simulink model "uncontrolled_group24"  (R2023b)
settings: Solver=ode5  StartTime=0.0  StopTime=333  FixedStep=0.1  RelTol=1e-3
values from neighbouring files (symbols this model uses):
  a = 6939    [Air_Drag_script.m]    (also in main.m = 6939.063; main_group24.m = 6939.063)
  A0 = eye(3)    [Air_Drag_script.m]    (also in main_group24.m)
  ARW = 0.15    [main_group24.m]
  c = 2.99792*10^8    (= 299792000)    [main.m]    (also in main_group24.m)
  e = 0    [Air_Drag_script.m]    (also in main.m = 0.001304; main_group24.m)
  G = [gn, gm, gvali, gsvi]    [main.m]    (also in main_group24.m)
  GyroSampleRate = 10    [main_group24.m]
  H = [hn, hm, hvali, hsvi]    [main.m]    (also in main_group24.m)
  i = deg2rad(97.5307)    [Air_Drag_script.m]    (also in main.m; main_group24.m)
  I_tot = [Ix 0 0; 0 Iy 0; 0 0 Iz]    [data_mass.m]    (also in main_group24.m)
  invI_tot = inv(I_tot)    [data_mass.m]    (also in main_group24.m)
  Ix = J(1,1)    [Air_Drag_script.m]    (also in data_mass.m = 0.0755003333333; main.m = 0.057749855; main_group24.m = 0.0755003333333)
  Iy = J(2,2)    [Air_Drag_script.m]    (also in data_mass.m = 0.0755003333333; main.m = 0.04143542; main_group24.m = 0.0755003333333)
  Iz = J(3,3)    [Air_Drag_script.m]    (also in data_mass.m = 0.055; main.m = 0.024624309; main_group24.m = 0.055)
  m = [0.1; 0.1; 0.1]    [main.m]    (also in main_group24.m)
  MB = [4; 0.1; 0.1; 0.3]    [main.m]    (also in main_group24.m)
  MMnoise = 15e-9*[1; 1; 1]    [main_group24.m]
  MMSampleRate = 1    [main_group24.m]
  mu = 3.98600433e+5    (= 398600.433)    [main.m]    (also in main_group24.m)
  n = 0.0011    [Air_Drag_script.m]    (also in main.m = sqrt(mu/a^3); main_group24.m = sqrt(mu/a^3))
  q0 = [ 1 1 1 1 ]'    [Air_Drag_script.m]    (also in main_group24.m = [0 0 0 1]')
  R_e = 6378    [main.m]    (also in main_group24.m)
  rho_air = 1.65e-13    [Air_Drag_script.m]
  rho_d_MB = 0.1    [main.m]    (also in main_group24.m)
  rho_d_SP = 0.1    [main.m]    (also in main_group24.m)
  rho_s_MB = 0.5    [main.m]    (also in main_group24.m)
  rho_s_SP = 0.1    [main.m]    (also in main_group24.m)
  RRW = 0.3    [main_group24.m]
  SP = [1; 0.3; 0.1; 0.01]    [main.m]    (also in main_group24.m = [0.25; 0.1; 0.3; 0.01])
  w0 = [0 0 0]'    [Air_Drag_script.m]    (also in main.m = [wx0; wy0; wz0]; main_group24.m = [wx0; wy0; wz0])
undefined symbols (not defined in the file or in its folder): Cd, H_0, n_E, P, pan1, pan2, rho_d_body, rho_d_sp, rho_s_body, rho_s_sp, s1, s2, s3, s4, s5, s6, v_rel
libraries: vrlib x40, simulink_extras x13, matrix_library x8, sharedutil x3, simulink x1
(part 1 of 4)
settings Model: Creator=lucag  LastModifiedBy=lucag
settings OptimizationCC: ReuseModelBlockBuffer=off

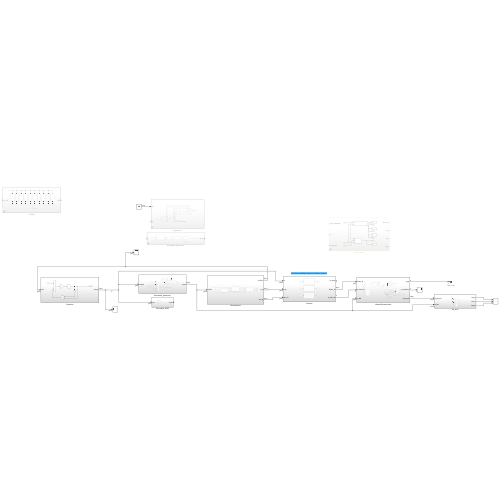
[thumbnail: Simulink's stored preview of the top-level diagram]
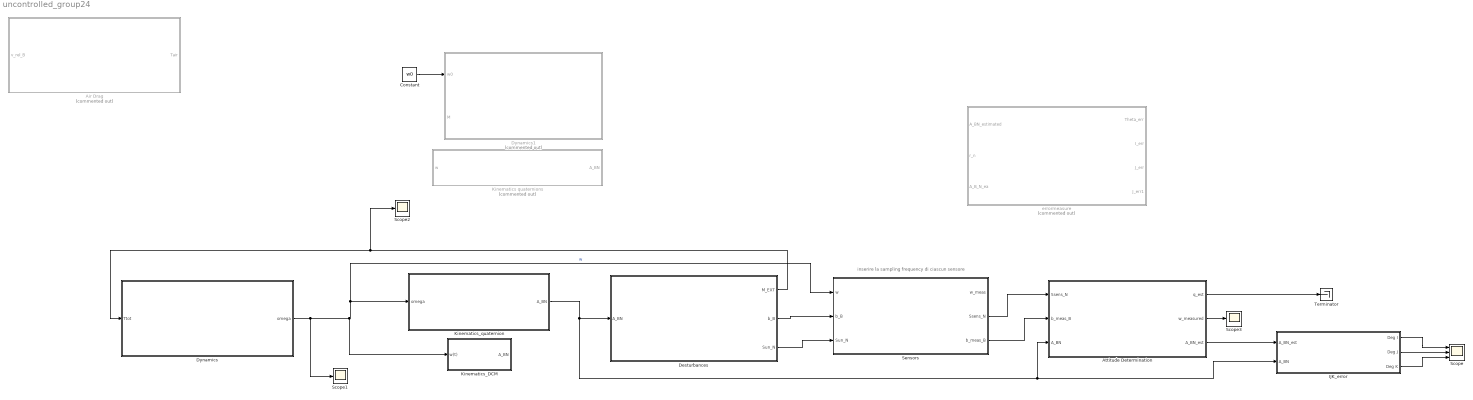
== system uncontrolled_group24 ==
  note: inserire la sampling frequency di ciascun sensore
  Air Drag : Subsystem  Commented=on
  Attitude Determination : Subsystem
  Constant : Constant  Value=w0  VectorParams1D=off
  Desturbances : Subsystem
  Dynamics : Subsystem
  Dynamics1 : Subsystem  Commented=on
  IJK_error : Subsystem
  Kinematics quaternions : Subsystem  Commented=on
  Kinematics_DCM : Subsystem
  Kinematics_quaternion : Subsystem
  Scope : Scope  NumInputPorts=3
  Scope1 : Scope
  Scope2 : Scope
  Scope3 : Scope
  Sensors : Subsystem
  Terminator : Terminator
  errormeasure : Subsystem  Commented=on
  wires:
  Desturbances/2(b_B) -> Sensors/2(b_B)
  Desturbances/3(Sun_N) -> Sensors/3(Sun_N)
  Sensors/3(b_meas_B) -> Attitude Determination/2(b_meas_B)
  Constant/1 -> Dynamics1/1(w0)
  Sensors/2(Ssens_N) -> Attitude Determination/1(Ssens_N)
  Dynamics/1(omega) -> Scope1/1, Kinematics_DCM/1(w(t)), Kinematics_quaternion/1(omega), Sensors/1(w)  "w"
  Attitude Determination/1(q_est) -> Terminator/1
  Desturbances/1(M_EXT) -> Dynamics/1(Ttot), Scope2/1
  Attitude Determination/2(w_measured) -> Scope3/1
  Kinematics_quaternion/1(A_BN) -> Attitude Determination/3(A_BN), IJK_error/2(A_BN), Desturbances/1(A_BN)
  Attitude Determination/3(A_BN_est) -> IJK_error/1(A_BN_est)
  IJK_error/2(Deg J) -> Scope/2
  IJK_error/1(Deg I) -> Scope/1
  IJK_error/3(Deg K) -> Scope/3

== system uncontrolled_group24/Air Drag ==
  v_rel_B : Inport
  Subsystem : Subsystem
  Subsystem1 : Subsystem
  Subsystem2 : Subsystem
  Subsystem3 : Subsystem
  Subsystem4 : Subsystem
  Subsystem5 : Subsystem
  Subsystem6 : Subsystem
  Subsystem7 : Subsystem
  Subsystem8 : Subsystem
  Subsystem9 : Subsystem
  Sum : Sum  Inputs=++++++++++
  Tair : Outport
  wires:
  v_rel_B/1 -> Subsystem1/1(v_rel_B), Subsystem2/1(v_rel_B), Subsystem3/1(v_rel_B), Subsystem4/1(v_rel_B), Subsystem5/1(v_rel_B), Subsystem6/1(v_rel_B), Subsystem7/1(v_rel_B), Subsystem8/1(v_rel_B), Subsystem9/1(v_rel_B), Subsystem/1(v_rel_B)
  Sum/1 -> Tair/1
  Subsystem/1(Pan1) -> Sum/1
  Subsystem1/1(Pan2) -> Sum/2
  Subsystem2/1(Pan3) -> Sum/3
  Subsystem3/1(Pan4) -> Sum/4
  Subsystem4/1(Pan5) -> Sum/5
  Subsystem5/1(Pan6) -> Sum/6
  Subsystem6/1(Ps1) -> Sum/7
  Subsystem7/1(Ps2) -> Sum/8
  Subsystem8/1(Ps3) -> Sum/9
  Subsystem9/1(Ps4) -> Sum/10

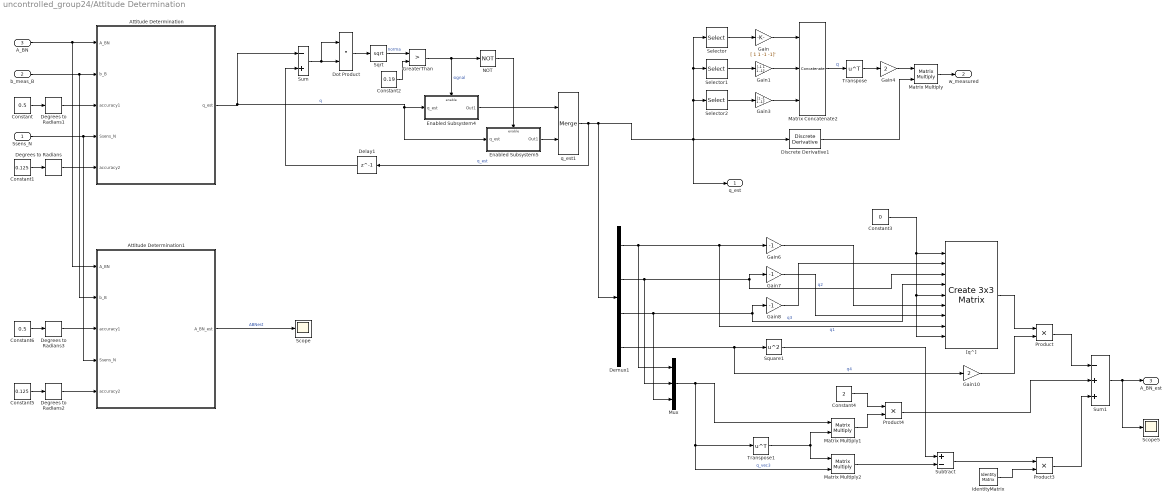
== system uncontrolled_group24/Attitude Determination ==
  Ssens_N : Inport
  b_meas_B : Inport  Port=2
  A_BN : Inport  Port=3
  Attitude Determination : MATLAB Function  TreatAsAtomicUnit=on
  Attitude Determination1 : MATLAB Function  TreatAsAtomicUnit=on
  Constant : Constant  Value=0.5
  Constant1 : Constant  Value=0.125
  Constant2 : Constant  Value=0.19
  Constant3 : Constant  Value=0
  Constant4 : Constant  Value=2
  Constant5 : Constant  Value=0.125
  Constant6 : Constant  Value=0.5
  Degrees to Radians{,1..3} (4 alike) : simulink_extras/Transformations/Degrees to Radians
  Delay1 : Delay  DelayLength=1  InitialCondition=q0
  Demux1 : Demux
  Discrete Derivative1 : simulink/Discrete/Discrete Derivative  gainval=1.0  ICPrevScaledInput=0  OutMin=[]  OutMax=[]  OutDataType=fixdt(1, 16)  OutScaling=2^-10  DoSatur=off
  Dot Product : DotProduct  OutDataTypeStr=Inherit: Inherit via internal rule
  Enabled Subsystem4 : Subsystem  TreatAsAtomicUnit=on
  Enabled Subsystem5 : Subsystem  TreatAsAtomicUnit=on
  Gain : Gain  Gain=[ 1 1 -1 -1]'
  Gain1 : Gain  Gain=[-1 1 1 -1]'
  Gain10 : Gain  Gain=2
  Gain3 : Gain  Gain=[1 -1 1 -1]'
  Gain4 : Gain  Gain=2
  Gain6 : Gain  Gain=-1
  Gain7 : Gain  Gain=-1
  Gain8 : Gain  Gain=-1
  GreaterThan : RelationalOperator  Operator=>  OutDataTypeStr=boolean  RndMeth=Simplest  InputSameDT=off
  IdentityMatrix : IdentityMatrix  OutputDimensions=3
  Matrix Concatenate2 : Concatenate  NumInputs=3  Mode=Multidimensional array  ConcatenateDimension=2
  Matrix Multiply : Product  Multiplication=Matrix(*)
  Matrix Multiply1 : Product  Multiplication=Matrix(*)
  Matrix Multiply2 : Product  Multiplication=Matrix(*)
  Mux : Mux  Inputs=3
  NOT : Logic  Operator=NOT  IconShape=distinctive  AllPortsSameDT=off  OutDataTypeStr=boolean
  Product : Product
  Product3 : Product
  Product4 : Product
  Scope : Scope
  Scope5 : Scope
  Selector : Selector  InputPortWidth=4  IndexOptions=Index vector (dialog)  Indices=[4 3 2 1]  OutputSizes=1
  Selector1 : Selector  InputPortWidth=4  IndexOptions=Index vector (dialog)  Indices=[3 4 1 2]  OutputSizes=1
  Selector2 : Selector  InputPortWidth=4  IndexOptions=Index vector (dialog)  Indices=[2 1 4 3]  OutputSizes=1
  Sqrt : Sqrt
  Square1 : Math  Operator=square
  Subtract : Sum  Inputs=+-
  Sum : Sum  Inputs=-+
  Sum1 : Sum  Inputs=-++
  Transpose : Math  Operator=transpose
  Transpose1 : Math  Operator=transpose
  "[q^]" : sharedutil/Create 3x3 Matrix  aMode=aMode
      settings: LibrarySourceBlock=aerolibutil/Create 3x3 Matrix
  q_est1 : Merge
  q_est : Outport
  w_measured : Outport  Port=2
  A_BN_est : Outport  Port=3
  wires:
  b_meas_B/1 -> Attitude Determination1/2(b_B), Attitude Determination/2(b_B)
  Ssens_N/1 -> Attitude Determination1/4(Ssens_N), Attitude Determination/4(Ssens_N)
  Constant1/1 -> Degrees to Radians/1
  Constant/1 -> Degrees to Radians1/1
  A_BN/1 -> Attitude Determination1/1(A_BN), Attitude Determination/1(A_BN)
  Gain1/1 -> Matrix Concatenate2/2
  Matrix Multiply/1 -> w_measured/1
  Gain4/1 -> Matrix Multiply/1
  Gain/1 -> Matrix Concatenate2/1
  Selector/1 -> Gain/1
  Selector2/1 -> Gain3/1
  Transpose/1 -> Gain4/1
  Discrete Derivative1/1 -> Matrix Multiply/2
  Matrix Concatenate2/1 -> Transpose/1  "Q"
  Selector1/1 -> Gain1/1
  Gain3/1 -> Matrix Concatenate2/3
  Degrees to Radians1/1 -> Attitude Determination/3(accuracy1)
  Degrees to Radians/1 -> Attitude Determination/5(accuracy2)
  q_est1/1 -> Demux1/1, q_est/1, Selector1/1, Selector/1, Selector2/1, Discrete Derivative1/1, Delay1/1  "q_est"
  GreaterThan/1 -> NOT/1, Enabled Subsystem4/Enable  "signal"
  Enabled Subsystem5/1(Out1) -> q_est1/2
  Sum/1 -> Dot Product/1, Dot Product/2
  Delay1/1 -> Sum/2
  NOT/1 -> Enabled Subsystem5/Enable
  Enabled Subsystem4/1(Out1) -> q_est1/1
  Constant2/1 -> GreaterThan/2
  Sqrt/1 -> GreaterThan/1  "norma"
  Dot Product/1 -> Sqrt/1
  Attitude Determination/1(q_est) -> Enabled Subsystem4/1(q_est), Enabled Subsystem5/1(q_est), Sum/1  "q"
  "[q^]"/1 -> Product/1
  Square1/1 -> Subtract/1
  Matrix Multiply1/1 -> Product4/2
  Gain10/1 -> Product/2
  Sum1/1 -> Scope5/1, A_BN_est/1
  Product/1 -> Sum1/1
  Gain8/1 -> "[q^]"/2
  Constant4/1 -> Product4/1
  Mux/1 -> Matrix Multiply1/1, Transpose1/1, Matrix Multiply2/2  "q_vec3"
  IdentityMatrix/1 -> Product3/2
  Transpose1/1 -> Matrix Multiply1/2, Matrix Multiply2/1
  Matrix Multiply2/1 -> Subtract/2
  Demux1/4 -> Gain10/1, Square1/1  "q4"
  Gain6/1 -> "[q^]"/6
  Demux1/2 -> Mux/2, Gain7/1, "[q^]"/3  "q2"
  Constant3/1 -> "[q^]"/5, "[q^]"/9, "[q^]"/1
  Gain7/1 -> "[q^]"/7
  Demux1/3 -> Mux/3, Gain8/1, "[q^]"/4  "q3"
  Product3/1 -> Sum1/3
  Product4/1 -> Sum1/2
  Demux1/1 -> Mux/1, Gain6/1, "[q^]"/8  "q1"
  Subtract/1 -> Product3/1
  Attitude Determination1/1(A_BN_est) -> Scope/1  "ABNest"
  Degrees to Radians2/1 -> Attitude Determination1/5(accuracy2)
  Constant5/1 -> Degrees to Radians2/1
  Degrees to Radians3/1 -> Attitude Determination1/3(accuracy1)
  Constant6/1 -> Degrees to Radians3/1

== system uncontrolled_group24/Desturbances ==
  A_BN : Inport
  External Torques : Subsystem
  Orbital Mechanics : Subsystem
  Relative Attitude : Subsystem
  M_EXT : Outport
  b_B : Outport  Port=2
  Sun_N : Outport  Port=3
  wires:
  Relative Attitude/1(A_BL.) -> External Torques/1(A_BL)
  Relative Attitude/2(r_L) -> External Torques/2(r_L)
  A_BN/1 -> External Torques/4(A_BN), Relative Attitude/1(A_BN_ideal)
  Orbital Mechanics/1(theta) -> Relative Attitude/2(theta)
  Orbital Mechanics/2(r_N) -> Relative Attitude/3(r_N)
  Orbital Mechanics/3(r) -> External Torques/3(r)
  External Torques/1(M_EXT) -> M_EXT/1
  External Torques/2(b_B) -> b_B/1
  External Torques/3(Sun_N) -> Sun_N/1

== system uncontrolled_group24/Dynamics ==
  note: omega
  Ttot : Inport
  Add : Sum
  Cross Product : vrlib/Utilities/Cross Product
  Gain : Gain  Gain=invI_tot  Multiplication=Matrix(K*u)
  Gain1 : Gain  Gain=I_tot  Multiplication=Matrix(K*u)
  Integrator3 : Integrator  InitialCondition=w0  AbsoluteTolerance=10^-7
  omega : Outport
  wires:
  Gain1/1 -> Cross Product/1
  Ttot/1 -> Add/1
  Cross Product/1 -> Add/2
  Integrator3/1 -> omega/1, Cross Product/2, Gain1/1
  Gain/1 -> Integrator3/1
  Add/1 -> Gain/1

== system uncontrolled_group24/Dynamics1 ==
  w0 : Inport
  M : Inport  Port=2
  Demux : Demux  Outputs=3
  Demux1 : Demux  Outputs=3
  Gain : Gain  Gain=(Iy-Iz)/Ix
  Gain1 : Gain  Gain=(Iz-Ix)/Iy
  Gain2 : Gain  Gain=(Ix-Iy)/Iz
  Sum : Sum  Inputs=|++
  Sum1 : Sum  Inputs=|++
  Sum2 : Sum  Inputs=|++
  Vector Concatenate : Concatenate  NumInputs=3  Mode=Multidimensional array
  XZ : Product
  YX : Product
  ZY : Product
  wx : Integrator  InitialConditionSource=external
  wy : Integrator  InitialConditionSource=external
  wz : Integrator  InitialConditionSource=external
  wires:
  XZ/1 -> Gain1/1
  Demux/2 -> wy/2  "wy0"
  wx/1 -> XZ/1, Vector Concatenate/1, YX/1
  w0/1 -> Demux/1
  wy/1 -> Vector Concatenate/2, YX/2, ZY/2
  Demux/1 -> wx/2  "wx0"
  wz/1 -> ZY/1, Vector Concatenate/3, XZ/2
  YX/1 -> Gain2/1
  Demux/3 -> wz/2  "wz0"
  ZY/1 -> Gain/1
  Vector Concatenate/1 -> ?
  Gain2/1 -> Sum2/1
  Gain1/1 -> Sum1/1
  Gain/1 -> Sum/1
  Sum/1 -> wx/1
  Sum1/1 -> wy/1
  Sum2/1 -> wz/1
  Demux1/1 -> Sum/2  "Mx"
  Demux1/2 -> Sum1/2  "My"
  Demux1/3 -> Sum2/2  "Mz"
  M/1 -> Demux1/1

== system uncontrolled_group24/IJK_error ==
  A_BN_est : Inport
  A_BN : Inport  Port=2
  I : Constant  Value=[1 0 0]'
  I_Error : Subsystem
  J : Constant  Value=[0 1 0]'
  J_Error : Subsystem
  K : Constant  Value=[0 0 1]'
  K_Error : Subsystem
  Deg I : Outport
  Deg J : Outport  Port=2
  Deg K : Outport  Port=3
  wires:
  J_Error/1(Deg J) -> Deg J/1
  J/1 -> J_Error/2(J)
  I_Error/1(Deg I) -> Deg I/1
  K_Error/1(Deg K) -> Deg K/1
  I/1 -> I_Error/2(I)
  K/1 -> K_Error/2(K)
  A_BN_est/1 -> J_Error/1(A_BN_est), K_Error/1(A_BN_est), I_Error/1(A_BN_est)
  A_BN/1 -> J_Error/3(A_BN), K_Error/3(A_BN), I_Error/3(A_BN)

== system uncontrolled_group24/Kinematics quaternions ==
  w : Inport
  A_matrix : Subsystem
  Create Omega Matrix : Subsystem
  Kinematics_quaternions : Subsystem
  Normalizer : Subsystem
  Subsystem : Subsystem  Commented=on
  w_at_matrix : Subsystem
  A_BN : Outport
  wires:
  Kinematics_quaternions/1(q_vect) -> A_matrix/1(q_vect)
  A_matrix/1(A_BN) -> Normalizer/1(A_BN)
  w/1 -> Create Omega Matrix/2(w), w_at_matrix/1(w(t))
  Create Omega Matrix/1(Omega) -> Kinematics_quaternions/1(Omega)  "Omega"
  w_at_matrix/1("[-w^]") -> Create Omega Matrix/1("[w^]")  "[-w^]"
  Normalizer/1(Out1) -> A_BN/1

== system uncontrolled_group24/Kinematics_DCM ==
  w(t) : Inport
  Constant : Constant  Value=0
  Constant1 : Constant  Value=0
  Constant2 : Constant  Value=0
  Demux : Demux  Outputs=3
  Integrator : Integrator  InitialCondition=A0
  Matrix Concatenate : Concatenate  NumInputs=3  Mode=Multidimensional array
  MatrixMultiply : Product  Multiplication=Matrix(*)
  Multiply{,1..3} (4 alike) : Gain  Gain=-1
  Mux : Mux  Inputs=3
  Mux1 : Mux  Inputs=3
  Mux2 : Mux  Inputs=3
  Reshape : Reshape  OutputDimensionality=Row vector (2-D)
  Reshape1 : Reshape  OutputDimensionality=Row vector (2-D)
  Reshape2 : Reshape  OutputDimensionality=Row vector (2-D)
  Scope : Scope
  Subsystem : Subsystem
  A_BN : Outport
  wires:
  w(t)/1 -> Demux/1  "omega"
  MatrixMultiply/1 -> Integrator/1  "dA_dt"
  Matrix Concatenate/1 -> Multiply3/1  "omega_hat"
  Constant/1 -> Mux/1
  Demux/3 -> Mux1/1, Multiply/1  "w_z"
  Multiply/1 -> Mux/2
  Demux/2 -> Mux/3, Multiply2/1  "w_y"
  Constant1/1 -> Mux1/2
  Demux/1 -> Mux2/2, Multiply1/1  "w_x"
  Multiply1/1 -> Mux1/3
  Constant2/1 -> Mux2/3
  Multiply2/1 -> Mux2/1
  Mux/1 -> Reshape/1
  Mux1/1 -> Reshape1/1
  Mux2/1 -> Reshape2/1
  Multiply3/1 -> MatrixMultiply/1
  Reshape/1 -> Matrix Concatenate/1
  Reshape1/1 -> Matrix Concatenate/2
  Reshape2/1 -> Matrix Concatenate/3
  Integrator/1 -> Subsystem/1(In1), MatrixMultiply/2  "A_BN"
  Subsystem/1(Out2) -> A_BN/1, Scope/1

== system uncontrolled_group24/Kinematics_quaternion ==
  omega : Inport
  Constant : Constant  Value=0
  Constant1 : Constant  Value=0
  Constant2 : Constant  Value=2
  Demux : Demux  Outputs=3
  Demux1 : Demux
  Divide : Product  Inputs=/*
  Dot Product : DotProduct  OutDataTypeStr=Inherit: Inherit via internal rule
  Gain{1..3,6..8} (6 alike) : Gain  Gain=-1
  Gain10 : Gain  Gain=2
  Gain9 : Gain  Gain=1/2
  IdentityMatrix : IdentityMatrix  OutputDimensions=3
  Integrator : Integrator  InitialCondition=[0 0 0 1]
  Matrix Multiply : Product  Multiplication=Matrix(*)
  Matrix Multiply1 : Product  Multiplication=Matrix(*)
  Matrix Multiply2 : Product  Multiplication=Matrix(*)
  Mux : Mux  Inputs=3
  OMEGA : Concatenate  NumInputs=16  Mode=Multidimensional array  ConcatenateDimension=2
  Product : Product
  Product3 : Product
  Product4 : Product
  Reshape : Reshape  OutputDimensionality=Customize  OutputDimensions=[4,4]
  Scope : Scope
  Scope5 : Scope
  Square Root2 : Sqrt
  Square1 : Math  Operator=square
  Subtract : Sum  Inputs=+-
  Sum : Sum  Inputs=-++
  Transpose : Math  Operator=transpose
  "[q^]" : sharedutil/Create 3x3 Matrix  aMode=aMode
      settings: LibrarySourceBlock=aerolibutil/Create 3x3 Matrix
  A_BN : Outport
  wires:
  Matrix Multiply/1 -> Gain9/1
  Square Root2/1 -> Divide/1
  Constant/1 -> OMEGA/16, OMEGA/11, OMEGA/6, OMEGA/1
  Integrator/1 -> Dot Product/1, Dot Product/2, Divide/2  "q"
  OMEGA/1 -> Reshape/1
  Constant1/1 -> "[q^]"/5, "[q^]"/9, "[q^]"/1
  Demux1/1 -> Mux/1, Gain6/1, "[q^]"/8  "q1"
  Demux1/2 -> Mux/2, Gain7/1, "[q^]"/3  "q2"
  Demux1/4 -> Gain10/1, Square1/1  "q4"
  Gain8/1 -> "[q^]"/2
  Gain6/1 -> "[q^]"/6
  Gain7/1 -> "[q^]"/7
  Transpose/1 -> Matrix Multiply1/2, Matrix Multiply2/1
  Gain10/1 -> Product/2
  "[q^]"/1 -> Product/1
  Square1/1 -> Subtract/1
  Matrix Multiply2/1 -> Subtract/2
  Divide/1 -> Scope/1, Demux1/1, Matrix Multiply/2  "q"
  Subtract/1 -> Product3/1
  IdentityMatrix/1 -> Product3/2
  Product/1 -> Sum/1
  Product3/1 -> Sum/3
  Constant2/1 -> Product4/1
  Matrix Multiply1/1 -> Product4/2
  Product4/1 -> Sum/2
  Demux1/3 -> Mux/3, Gain8/1, "[q^]"/4  "q3"
  Mux/1 -> Matrix Multiply1/1, Transpose/1, Matrix Multiply2/2  "q_vec3"
  Sum/1 -> Scope5/1, A_BN/1
  Dot Product/1 -> Square Root2/1
  Reshape/1 -> Matrix Multiply/1
  Gain9/1 -> Integrator/1  "q_dot"
  omega/1 -> Demux/1
  Demux/1 -> OMEGA/7, OMEGA/4, Gain2/1  "wx"
  Demux/2 -> OMEGA/8, OMEGA/9, Gain3/1  "wy"
  Demux/3 -> OMEGA/2, OMEGA/12, Gain1/1  "wz"
  Gain3/1 -> OMEGA/3, OMEGA/14
  Gain1/1 -> OMEGA/5, OMEGA/15
  Gain2/1 -> OMEGA/13, OMEGA/10

== system uncontrolled_group24/Sensors ==
  w : Inport
  b_B : Inport  Port=2
  Sun_N : Inport  Port=3
  Gyroscope : Subsystem
  Magnetometer : Subsystem
  Sun Sensor : Subsystem
  w_meas : Outport
  Ssens_N : Outport  Port=2
  b_meas_B : Outport  Port=3
  wires:
  w/1 -> Gyroscope/1(w)
  Gyroscope/1(w_meas) -> w_meas/1
  Sun Sensor/1(Ssens_N) -> Ssens_N/1
  Sun_N/1 -> Sun Sensor/1(Sun_N)
  b_B/1 -> Magnetometer/1(b_B)
  Magnetometer/1(b_meas_B) -> b_meas_B/1

== system uncontrolled_group24/errormeasure ==
  A_BN_estimated : Inport
  r_n : Inport  Port=2
  A_B_N_ea : Inport  Port=3
  IJK_error : Subsystem
  To Workspace : ToWorkspace  VariableName=Theta_err  SampleTime=-1
  To Workspace1 : ToWorkspace  VariableName=I_err  SampleTime=-1
  To Workspace2 : ToWorkspace  VariableName=J_err  SampleTime=-1
  To Workspace3 : ToWorkspace  VariableName=K_Error  SampleTime=-1
  r_n_Error : Subsystem
  Theta_err : Outport
  I_err : Outport  Port=2
  J_err : Outport  Port=3
  J_err1 : Outport  Port=4
  wires:
  A_B_N_ea/1 -> r_n_Error/3(A_B_N_ea), IJK_error/2(A_B_N_ea)
  IJK_error/2(Degrees out1) -> J_err/1, To Workspace2/1
  r_n/1 -> r_n_Error/2(r_n)
  A_BN_estimated/1 -> r_n_Error/1(A_BN_estimated), IJK_error/1(A_BN_estimated)
  r_n_Error/1(Degrees out) -> Theta_err/1, To Workspace/1
  IJK_error/1(Degrees out) -> To Workspace1/1, I_err/1
  IJK_error/3(Degrees out2) -> To Workspace3/1, J_err1/1

== system uncontrolled_group24/Air Drag/Subsystem ==
  v_rel_B : Inport
  Constant : Constant  Value=-0.5
  Constant1 : Constant  Value=s1.n
  Constant2 : Constant  Value=s1.r
  Constant3 : Constant  Value=s1.A
  Cross Product2 : vrlib/Utilities/Cross Product
  Dot Product1 : DotProduct  OutDataTypeStr=Inherit: Inherit via internal rule
  Gain : Gain  Gain=rho_air
  Gain1 : Gain  Gain=0
  Gain2 : Gain  Gain=Cd
  Gain3 : Gain  Gain=v_rel^2
  Product : Product  Inputs=4
  Switch1 : Switch  Criteria=u2 > Threshold  SaturateOnIntegerOverflow=off  InputSameDT=off
  Pan1 : Outport
  wires:
  Constant2/1 -> Cross Product2/1
  Gain1/1 -> Switch1/3
  Dot Product1/1 -> Gain1/1, Switch1/2, Switch1/1
  Constant3/1 -> Product/2
  Product/1 -> Cross Product2/2
  Switch1/1 -> Product/4
  v_rel_B/1 -> Dot Product1/1, Product/3
  Gain3/1 -> Product/1
  Gain/1 -> Gain2/1
  Constant/1 -> Gain/1
  Cross Product2/1 -> Pan1/1
  Constant1/1 -> Dot Product1/2
  Gain2/1 -> Gain3/1

== system uncontrolled_group24/Air Drag/Subsystem1 ==
  v_rel_B : Inport
  Constant : Constant  Value=-0.5
  Constant1 : Constant  Value=s1.n
  Constant2 : Constant  Value=s1.r
  Constant3 : Constant  Value=s1.A
  Cross Product2 : vrlib/Utilities/Cross Product
  Dot Product1 : DotProduct  OutDataTypeStr=Inherit: Inherit via internal rule
  Gain : Gain  Gain=rho_air
  Gain1 : Gain  Gain=0
  Gain2 : Gain  Gain=Cd
  Gain3 : Gain  Gain=v_rel^2
  Product : Product  Inputs=4
  Switch1 : Switch  Criteria=u2 > Threshold  SaturateOnIntegerOverflow=off  InputSameDT=off
  Pan2 : Outport
  wires:
  Gain2/1 -> Gain3/1
  Constant1/1 -> Dot Product1/2
  Cross Product2/1 -> Pan2/1
  Constant/1 -> Gain/1
  Gain/1 -> Gain2/1
  Gain3/1 -> Product/1
  v_rel_B/1 -> Product/3, Dot Product1/1
  Switch1/1 -> Product/4
  Product/1 -> Cross Product2/2
  Constant3/1 -> Product/2
  Dot Product1/1 -> Switch1/1, Switch1/2, Gain1/1
  Gain1/1 -> Switch1/3
  Constant2/1 -> Cross Product2/1

== system uncontrolled_group24/Air Drag/Subsystem2 ==
  v_rel_B : Inport
  Constant : Constant  Value=-0.5
  Constant1 : Constant  Value=s1.n
  Constant2 : Constant  Value=s1.r
  Constant3 : Constant  Value=s1.A
  Cross Product2 : vrlib/Utilities/Cross Product
  Dot Product1 : DotProduct  OutDataTypeStr=Inherit: Inherit via internal rule
  Gain : Gain  Gain=rho_air
  Gain1 : Gain  Gain=0
  Gain2 : Gain  Gain=Cd
  Gain3 : Gain  Gain=v_rel^2
  Product : Product  Inputs=4
  Switch1 : Switch  Criteria=u2 > Threshold  SaturateOnIntegerOverflow=off  InputSameDT=off
  Pan3 : Outport
  wires:
  Constant2/1 -> Cross Product2/1
  Gain1/1 -> Switch1/3
  Dot Product1/1 -> Gain1/1, Switch1/2, Switch1/1
  Constant3/1 -> Product/2
  Product/1 -> Cross Product2/2
  Switch1/1 -> Product/4
  v_rel_B/1 -> Dot Product1/1, Product/3
  Gain3/1 -> Product/1
  Gain/1 -> Gain2/1
  Constant/1 -> Gain/1
  Cross Product2/1 -> Pan3/1
  Constant1/1 -> Dot Product1/2
  Gain2/1 -> Gain3/1

== system uncontrolled_group24/Air Drag/Subsystem3 ==
  v_rel_B : Inport
  Constant : Constant  Value=-0.5
  Constant1 : Constant  Value=s1.n
  Constant2 : Constant  Value=s1.r
  Constant3 : Constant  Value=s1.A
  Cross Product2 : vrlib/Utilities/Cross Product
  Dot Product1 : DotProduct  OutDataTypeStr=Inherit: Inherit via internal rule
  Gain : Gain  Gain=rho_air
  Gain1 : Gain  Gain=0
  Gain2 : Gain  Gain=Cd
  Gain3 : Gain  Gain=v_rel^2
  Product : Product  Inputs=4
  Switch1 : Switch  Criteria=u2 > Threshold  SaturateOnIntegerOverflow=off  InputSameDT=off
  Pan4 : Outport
  wires:
  Gain2/1 -> Gain3/1
  Constant1/1 -> Dot Product1/2
  Cross Product2/1 -> Pan4/1
  Constant/1 -> Gain/1
  Gain/1 -> Gain2/1
  Gain3/1 -> Product/1
  v_rel_B/1 -> Product/3, Dot Product1/1
  Switch1/1 -> Product/4
  Product/1 -> Cross Product2/2
  Constant3/1 -> Product/2
  Dot Product1/1 -> Switch1/1, Switch1/2, Gain1/1
  Gain1/1 -> Switch1/3
  Constant2/1 -> Cross Product2/1

== system uncontrolled_group24/Air Drag/Subsystem4 ==
  v_rel_B : Inport
  Constant : Constant  Value=-0.5
  Constant1 : Constant  Value=s1.n
  Constant2 : Constant  Value=s1.r
  Constant3 : Constant  Value=s1.A
  Cross Product2 : vrlib/Utilities/Cross Product
  Dot Product1 : DotProduct  OutDataTypeStr=Inherit: Inherit via internal rule
  Gain : Gain  Gain=rho_air
  Gain1 : Gain  Gain=0
  Gain2 : Gain  Gain=Cd
  Gain3 : Gain  Gain=v_rel^2
  Product : Product  Inputs=4
  Switch1 : Switch  Criteria=u2 > Threshold  SaturateOnIntegerOverflow=off  InputSameDT=off
  Pan5 : Outport
  wires:
  Constant2/1 -> Cross Product2/1
  Gain1/1 -> Switch1/3
  Dot Product1/1 -> Gain1/1, Switch1/2, Switch1/1
  Constant3/1 -> Product/2
  Product/1 -> Cross Product2/2
  Switch1/1 -> Product/4
  v_rel_B/1 -> Dot Product1/1, Product/3
  Gain3/1 -> Product/1
  Gain/1 -> Gain2/1
  Constant/1 -> Gain/1
  Cross Product2/1 -> Pan5/1
  Constant1/1 -> Dot Product1/2
  Gain2/1 -> Gain3/1

== system uncontrolled_group24/Air Drag/Subsystem5 ==
  v_rel_B : Inport
  Constant : Constant  Value=-0.5
  Constant1 : Constant  Value=s1.n
  Constant2 : Constant  Value=s1.r
  Constant3 : Constant  Value=s1.A
  Cross Product2 : vrlib/Utilities/Cross Product
  Dot Product1 : DotProduct  OutDataTypeStr=Inherit: Inherit via internal rule
  Gain : Gain  Gain=rho_air
  Gain1 : Gain  Gain=0
  Gain2 : Gain  Gain=Cd
  Gain3 : Gain  Gain=v_rel^2
  Product : Product  Inputs=4
  Switch1 : Switch  Criteria=u2 > Threshold  SaturateOnIntegerOverflow=off  InputSameDT=off
  Pan6 : Outport
  wires:
  Constant2/1 -> Cross Product2/1
  Gain1/1 -> Switch1/3
  Dot Product1/1 -> Gain1/1, Switch1/2, Switch1/1
  Constant3/1 -> Product/2
  Product/1 -> Cross Product2/2
  Switch1/1 -> Product/4
  v_rel_B/1 -> Dot Product1/1, Product/3
  Gain3/1 -> Product/1
  Gain/1 -> Gain2/1
  Constant/1 -> Gain/1
  Cross Product2/1 -> Pan6/1
  Constant1/1 -> Dot Product1/2
  Gain2/1 -> Gain3/1

== system uncontrolled_group24/Air Drag/Subsystem6 ==
  v_rel_B : Inport
  Constant : Constant  Value=-0.5
  Constant1 : Constant  Value=s1.n
  Constant2 : Constant  Value=s1.r
  Constant3 : Constant  Value=s1.A
  Cross Product2 : vrlib/Utilities/Cross Product
  Dot Product1 : DotProduct  OutDataTypeStr=Inherit: Inherit via internal rule
  Gain : Gain  Gain=rho_air
  Gain1 : Gain  Gain=0
  Gain2 : Gain  Gain=Cd
  Gain3 : Gain  Gain=v_rel^2
  Product : Product  Inputs=4
  Switch1 : Switch  Criteria=u2 > Threshold  SaturateOnIntegerOverflow=off  InputSameDT=off
  Ps1 : Outport
  wires:
  Gain2/1 -> Gain3/1
  Constant1/1 -> Dot Product1/2
  Cross Product2/1 -> Ps1/1
  Constant/1 -> Gain/1
  Gain/1 -> Gain2/1
  Gain3/1 -> Product/1
  v_rel_B/1 -> Product/3, Dot Product1/1
  Switch1/1 -> Product/4
  Product/1 -> Cross Product2/2
  Constant3/1 -> Product/2
  Dot Product1/1 -> Switch1/1, Switch1/2, Gain1/1
  Gain1/1 -> Switch1/3
  Constant2/1 -> Cross Product2/1

== system uncontrolled_group24/Air Drag/Subsystem7 ==
  v_rel_B : Inport
  Constant : Constant  Value=-0.5
  Constant1 : Constant  Value=s1.n
  Constant2 : Constant  Value=s1.r
  Constant3 : Constant  Value=s1.A
  Cross Product2 : vrlib/Utilities/Cross Product
  Dot Product1 : DotProduct  OutDataTypeStr=Inherit: Inherit via internal rule
  Gain : Gain  Gain=rho_air
  Gain1 : Gain  Gain=0
  Gain2 : Gain  Gain=Cd
  Gain3 : Gain  Gain=v_rel^2
  Product : Product  Inputs=4
  Switch1 : Switch  Criteria=u2 > Threshold  SaturateOnIntegerOverflow=off  InputSameDT=off
  Ps2 : Outport
  wires:
  Constant2/1 -> Cross Product2/1
  Gain1/1 -> Switch1/3
  Dot Product1/1 -> Gain1/1, Switch1/2, Switch1/1
  Constant3/1 -> Product/2
  Product/1 -> Cross Product2/2
  Switch1/1 -> Product/4
  v_rel_B/1 -> Dot Product1/1, Product/3
  Gain3/1 -> Product/1
  Gain/1 -> Gain2/1
  Constant/1 -> Gain/1
  Cross Product2/1 -> Ps2/1
  Constant1/1 -> Dot Product1/2
  Gain2/1 -> Gain3/1

== system uncontrolled_group24/Air Drag/Subsystem8 ==
  v_rel_B : Inport
  Constant : Constant  Value=-0.5
  Constant1 : Constant  Value=s1.n
  Constant2 : Constant  Value=s1.r
  Constant3 : Constant  Value=s1.A
  Cross Product2 : vrlib/Utilities/Cross Product
  Dot Product1 : DotProduct  OutDataTypeStr=Inherit: Inherit via internal rule
  Gain : Gain  Gain=rho_air
  Gain1 : Gain  Gain=0
  Gain2 : Gain  Gain=Cd
  Gain3 : Gain  Gain=v_rel^2
  Product : Product  Inputs=4
  Switch1 : Switch  Criteria=u2 > Threshold  SaturateOnIntegerOverflow=off  InputSameDT=off
  Ps3 : Outport
  wires:
  Gain2/1 -> Gain3/1
  Constant1/1 -> Dot Product1/2
  Cross Product2/1 -> Ps3/1
  Constant/1 -> Gain/1
  Gain/1 -> Gain2/1
  Gain3/1 -> Product/1
  v_rel_B/1 -> Product/3, Dot Product1/1
  Switch1/1 -> Product/4
  Product/1 -> Cross Product2/2
  Constant3/1 -> Product/2
  Dot Product1/1 -> Switch1/1, Switch1/2, Gain1/1
  Gain1/1 -> Switch1/3
  Constant2/1 -> Cross Product2/1

== system uncontrolled_group24/Air Drag/Subsystem9 ==
  v_rel_B : Inport
  Constant : Constant  Value=-0.5
  Constant1 : Constant  Value=s1.n
  Constant2 : Constant  Value=s1.r
  Constant3 : Constant  Value=s1.A
  Cross Product2 : vrlib/Utilities/Cross Product
  Dot Product1 : DotProduct  OutDataTypeStr=Inherit: Inherit via internal rule
  Gain : Gain  Gain=rho_air
  Gain1 : Gain  Gain=0
  Gain2 : Gain  Gain=Cd
  Gain3 : Gain  Gain=v_rel^2
  Product : Product  Inputs=4
  Switch1 : Switch  Criteria=u2 > Threshold  SaturateOnIntegerOverflow=off  InputSameDT=off
  Ps4 : Outport
  wires:
  Constant2/1 -> Cross Product2/1
  Gain1/1 -> Switch1/3
  Dot Product1/1 -> Gain1/1, Switch1/2, Switch1/1
  Constant3/1 -> Product/2
  Product/1 -> Cross Product2/2
  Switch1/1 -> Product/4
  v_rel_B/1 -> Dot Product1/1, Product/3
  Gain3/1 -> Product/1
  Gain/1 -> Gain2/1
  Constant/1 -> Gain/1
  Cross Product2/1 -> Ps4/1
  Constant1/1 -> Dot Product1/2
  Gain2/1 -> Gain3/1

== system uncontrolled_group24/Attitude Determination/Enabled Subsystem4 ==
  q_est : Inport
  Enable : EnablePort
  Gain : Gain  Gain=-1
  Out1 : Outport
  wires:
  q_est/1 -> Gain/1
  Gain/1 -> Out1/1

== system uncontrolled_group24/Attitude Determination/Enabled Subsystem5 ==
  q_est : Inport
  Enable : EnablePort
  Out1 : Outport
  wires:
  q_est/1 -> Out1/1

== system uncontrolled_group24/Desturbances/External Torques ==
  A_BL : Inport
  r_L : Inport  Port=2
  r : Inport  Port=3
  A_BN : Inport  Port=4
  Constant : Constant  Value=MB
  Constant1 : Constant  Value=SP
  M_GG : Subsystem
  Mag field senza fcn : Subsystem  Commented=on
  Magnetic field : Subsystem
  SRP con frecce : Subsystem  Commented=on
  Solar radiation : Subsystem
  Sum of Elements : Sum  Inputs=+++
  To Workspace : ToWorkspace  VariableName=M_GG  SaveFormat=Timeseries  SampleTime=-1
  To Workspace1 : ToWorkspace  VariableName=M_SRP  SaveFormat=Timeseries  SampleTime=-1
  To Workspace2 : ToWorkspace  VariableName=M_MAG  SaveFormat=Timeseries  SampleTime=-1
  M_EXT : Outport
  b_B : Outport  Port=2
  Sun_N : Outport  Port=3
  wires:
  r/1 -> M_GG/2(r)
  Constant/1 -> Solar radiation/2(MB)
  Constant1/1 -> Solar radiation/3(SP)
  A_BN/1 -> Solar radiation/1(A_BN), Magnetic field/2(A_BN)
  Magnetic field/1(M_MAG) -> Sum of Elements/3, To Workspace2/1
  Sum of Elements/1 -> M_EXT/1
  A_BL/1 -> M_GG/1(A_BL)
  r_L/1 -> Magnetic field/1(r_L)
  M_GG/1(M_GG1) -> Sum of Elements/1, To Workspace/1
  Solar radiation/1(T_SRP) -> To Workspace1/1, Sum of Elements/2
  Magnetic field/2(b_B) -> b_B/1
  Solar radiation/2(Sun_N) -> Sun_N/1

== system uncontrolled_group24/Desturbances/Orbital Mechanics ==
  Sat Position magnitude : Subsystem
  Sat True Anomaly : Subsystem
  Sat position vector in inertial frame : Subsystem
  Scope : Scope
  theta : Outport
  r_N : Outport  Port=2
  r : Outport  Port=3
  wires:
  Sat True Anomaly/1(theta) -> Sat position vector in inertial frame/2(theta), theta/1, Sat Position magnitude/1(theta)  "theta"
  Sat Position magnitude/1(r) -> Scope/1, r/1, Sat position vector in inertial frame/1(r)
  Sat position vector in inertial frame/1(r_N) -> r_N/1  "r_N"

== system uncontrolled_group24/Desturbances/Relative Attitude ==
  A_BN_ideal : Inport
  theta : Inport  Port=2
  r_N : Inport  Port=3
  A_BL : Subsystem
  A_LN : Subsystem
  MatrixMultiply : Product  Multiplication=Matrix(*)
  A_BL. : Outport
  r_L : Outport  Port=2
  wires:
  A_LN/1(A_LN) -> MatrixMultiply/1, A_BL/2(A_LN)
  theta/1 -> A_LN/1(theta)
  A_BN_ideal/1 -> A_BL/1(A_BN)
  A_BL/1(A_BL) -> A_BL./1
  r_N/1 -> MatrixMultiply/2
  MatrixMultiply/1 -> r_L/1

== system uncontrolled_group24/IJK_error/I_Error ==
  A_BN_est : Inport
  I : Inport  Port=2
  A_BN : Inport  Port=3
  Acos : Trigonometry  Operator=acos
  Dot Product : DotProduct  OutDataTypeStr=Inherit: Inherit via internal rule
  MatrixMultiply : Product  Multiplication=Matrix(*)
  MatrixMultiply1 : Product  Multiplication=Matrix(*)
  Normalize Vector : vrlib/Utilities/Normalize Vector  maxzero=0
  Normalize Vector1 : vrlib/Utilities/Normalize Vector  maxzero=0
  Radians to Degrees : simulink_extras/Transformations/Radians to Degrees
  Deg I : Outport
  wires:
  MatrixMultiply1/1 -> Normalize Vector/1
  Dot Product/1 -> Acos/1
  I/1 -> MatrixMultiply1/2, MatrixMultiply/2
  Normalize Vector1/1 -> Dot Product/2
  Normalize Vector/1 -> Dot Product/1
  Acos/1 -> Radians to Degrees/1
  A_BN_est/1 -> MatrixMultiply1/1
  MatrixMultiply/1 -> Normalize Vector1/1
  A_BN/1 -> MatrixMultiply/1
  Radians to Degrees/1 -> Deg I/1

== system uncontrolled_group24/IJK_error/J_Error ==
  A_BN_est : Inport
  J : Inport  Port=2
  A_BN : Inport  Port=3
  Acos : Trigonometry  Operator=acos
  Dot Product : DotProduct  OutDataTypeStr=Inherit: Inherit via internal rule
  MatrixMultiply : Product  Multiplication=Matrix(*)
  MatrixMultiply1 : Product  Multiplication=Matrix(*)
  Normalize Vector : vrlib/Utilities/Normalize Vector  maxzero=0
  Normalize Vector1 : vrlib/Utilities/Normalize Vector  maxzero=0
  Radians to Degrees : simulink_extras/Transformations/Radians to Degrees
  Deg J : Outport
  wires:
  MatrixMultiply1/1 -> Normalize Vector/1
  Dot Product/1 -> Acos/1
  J/1 -> MatrixMultiply1/2, MatrixMultiply/2
  Normalize Vector1/1 -> Dot Product/2
  Normalize Vector/1 -> Dot Product/1
  Acos/1 -> Radians to Degrees/1
  A_BN_est/1 -> MatrixMultiply1/1
  MatrixMultiply/1 -> Normalize Vector1/1
  A_BN/1 -> MatrixMultiply/1
  Radians to Degrees/1 -> Deg J/1

== system uncontrolled_group24/IJK_error/K_Error ==
  A_BN_est : Inport
  K : Inport  Port=2
  A_BN : Inport  Port=3
  Acos : Trigonometry  Operator=acos
  Dot Product : DotProduct  OutDataTypeStr=Inherit: Inherit via internal rule
  MatrixMultiply : Product  Multiplication=Matrix(*)
  MatrixMultiply1 : Product  Multiplication=Matrix(*)
  Normalize Vector : vrlib/Utilities/Normalize Vector  maxzero=0
  Normalize Vector1 : vrlib/Utilities/Normalize Vector  maxzero=0
  Radians to Degrees : simulink_extras/Transformations/Radians to Degrees
  Deg K : Outport
  wires:
  MatrixMultiply1/1 -> Normalize Vector/1
  Dot Product/1 -> Acos/1
  K/1 -> MatrixMultiply1/2, MatrixMultiply/2
  Normalize Vector1/1 -> Dot Product/2
  Normalize Vector/1 -> Dot Product/1
  Acos/1 -> Radians to Degrees/1
  A_BN_est/1 -> MatrixMultiply1/1
  MatrixMultiply/1 -> Normalize Vector1/1
  A_BN/1 -> MatrixMultiply/1
  Radians to Degrees/1 -> Deg K/1

== system uncontrolled_group24/Kinematics quaternions/A_matrix ==
  q_vect : Inport
  Add : Sum  Inputs=++-
  Constant : Constant  Value=0
  Constant1 : Constant  Value=0
  Constant2 : Constant  Value=0
  Demux : Demux
  I : Constant  Value=eye(3)
  Matrix Concatenate : Concatenate  NumInputs=3  Mode=Multidimensional array
  MatrixMultiply : Product  Multiplication=Matrix(*)
  MatrixMultiply1 : Product
  MatrixMultiply2 : Product  Multiplication=Matrix(*)
  MatrixMultiply3 : Product
  Multiply : Gain  Gain=-1
  Multiply1 : Gain  Gain=-1
  Multiply2 : Gain  Gain=-1
  Multiply3 : Gain  Gain=2
  Multiply4 : Gain  Gain=2
  Mux{,1..3} (4 alike) : Mux  Inputs=3
  Reshape : Reshape  OutputDimensionality=Row vector (2-D)
  Reshape1 : Reshape  OutputDimensionality=Row vector (2-D)
  Reshape2 : Reshape  OutputDimensionality=Row vector (2-D)
  Square : Math  Operator=square
  Subtract : Sum  Inputs=-+
  Transpose : Math  Operator=transpose
  A_BN : Outport
  wires:
  q_vect/1 -> Demux/1
  Demux/1 -> Mux3/1, Mux2/2, Multiply1/1  "q1"
  Demux/2 -> Mux3/2, Mux/3, Multiply2/1  "q2"
  Demux/3 -> Mux3/3, Multiply/1, Mux1/1  "q3"
  Demux/4 -> Square/1, Multiply4/1  "q4"
  Mux/1 -> Reshape/1
  Reshape/1 -> Matrix Concatenate/1
  Mux1/1 -> Reshape1/1
  Mux2/1 -> Reshape2/1
  Reshape1/1 -> Matrix Concatenate/2
  Reshape2/1 -> Matrix Concatenate/3
  Multiply/1 -> Mux/2
  Constant1/1 -> Mux1/2
  Multiply1/1 -> Mux1/3
  Multiply2/1 -> Mux2/1
  Constant2/1 -> Mux2/3
  Matrix Concatenate/1 -> MatrixMultiply3/2  "q_hat"
  Mux3/1 -> MatrixMultiply2/1, Transpose/1, MatrixMultiply/2  "q_bar"
  Transpose/1 -> MatrixMultiply2/2, MatrixMultiply/1
  Square/1 -> Subtract/2
  MatrixMultiply/1 -> Subtract/1
  Subtract/1 -> MatrixMultiply1/1
  I/1 -> MatrixMultiply1/2
  MatrixMultiply2/1 -> Multiply3/1
  Multiply4/1 -> MatrixMultiply3/1
  Multiply3/1 -> Add/1
  MatrixMultiply1/1 -> Add/2
  MatrixMultiply3/1 -> Add/3
  Add/1 -> A_BN/1
  Constant/1 -> Mux/1

== system uncontrolled_group24/Kinematics quaternions/Create Omega Matrix ==
  "[w^]" : Inport
  w : Inport  Port=2
  " Col added" : Concatenate  Mode=Multidimensional array  ConcatenateDimension=2
  " Row added" : Concatenate  Mode=Multidimensional array
  Constant : Constant  Value=0
  Gain : Gain  Gain=-1
  Transpose : Math  Operator=transpose
  Vector Concatenate : Concatenate
  Omega : Outport
  wires:
  w/1 -> Transpose/1, Vector Concatenate/1
  Constant/1 -> Vector Concatenate/2
  Transpose/1 -> Gain/1
  "[w^]"/1 -> " Row added"/1
  " Row added"/1 -> " Col added"/1
  Vector Concatenate/1 -> " Col added"/2
  Gain/1 -> " Row added"/2
  " Col added"/1 -> Omega/1

== system uncontrolled_group24/Kinematics quaternions/Kinematics_quaternions ==
  Omega : Inport
  Constant : Constant  Value=q0  VectorParams1D=off
  Gain : Gain  Gain=0.5
  Integrator : Integrator  InitialConditionSource=external  InitialCondition=q0
  Omega*q(t) : Product  Multiplication=Matrix(*)
  Scope : Scope
  q_vect : Outport
  wires:
  Gain/1 -> Scope/1, q_vect/1, Integrator/1
  Integrator/1 -> Omega*q(t)/2  "q(t)"
  Omega*q(t)/1 -> Gain/1
  Omega/1 -> Omega*q(t)/1
  Constant/1 -> Integrator/2

== system uncontrolled_group24/Kinematics quaternions/Normalizer ==
  A_BN : Inport
  Gain : Gain  Gain=1.5
  Gain1 : Gain  Gain=0.5
  MatrixMultiply : Product  Multiplication=Matrix(*)
  MatrixMultiply1 : Product  Multiplication=Matrix(*)
  Sum : Sum  Inputs=+-
  Transpose : matrix_library/Transpose
  Out1 : Outport
  wires:
  A_BN/1 -> Transpose/1, MatrixMultiply/1, Gain/1, MatrixMultiply1/2
  Gain/1 -> Sum/1
  Sum/1 -> Out1/1
  Transpose/1 -> MatrixMultiply/2
  MatrixMultiply/1 -> MatrixMultiply1/1
  MatrixMultiply1/1 -> Gain1/1
  Gain1/1 -> Sum/2

== system uncontrolled_group24/Kinematics quaternions/Subsystem ==
  q_vect : Inport
  Demux : Demux
  From{,1..5} (6 alike) : From
  Goto{,1..8} (9 alike) : Goto
  Square{,1..3} (4 alike) : Math  Operator=square
  q1 q2 : Product
  q1 q3 : Product
  q1 q4 : Product
  q2 q4 : Product
  q3 q4 : Product
  Out1 : Outport
  wires:
  q_vect/1 -> Demux/1
  Demux/1 -> q1 q4/1, Square/1, q1 q3/1, q1 q2/1  "q1"
  Demux/2 -> Square1/1, q1 q2/2  "q2"
  Demux/3 -> q3 q4/2, Square2/1, q1 q3/2  "q3"
  Demux/4 -> q1 q4/2, q3 q4/1, Square3/1  "q4"
  q1 q2/1 -> Goto/1
  q1 q3/1 -> Goto1/1
  Square/1 -> Goto2/1
  Square1/1 -> Goto3/1
  Square2/1 -> Goto4/1
  Square3/1 -> Goto5/1
  q3 q4/1 -> Goto6/1
  q2 q4/1 -> Goto7/1
  q1 q4/1 -> Goto8/1

== system uncontrolled_group24/Kinematics quaternions/w_at_matrix ==
  w(t) : Inport
  Constant : Constant  Value=0  VectorParams1D=off
  Constant1 : Constant  Value=0
  Constant2 : Constant  Value=0
  Demux : Demux  Outputs=3
  Gain3 : Gain  Gain=-1
  Gain4 : Gain  Gain=-1
  Gain5 : Gain  Gain=-1
  Matrix Concatenate1 : Concatenate  NumInputs=3  Mode=Multidimensional array  ConcatenateDimension=2
  Mux1 : Mux  Inputs=3
  Mux2 : Mux  Inputs=3
  Mux3 : Mux  Inputs=3
  "[-w^]" : Outport
  wires:
  Demux/2 -> Mux1/3, Gain5/1  "wy"
  Gain3/1 -> Mux1/2
  Matrix Concatenate1/1 -> "[-w^]"/1
  Constant2/1 -> Mux3/3
  Demux/3 -> Mux2/1, Gain3/1  "wz"
  Constant1/1 -> Mux2/2
  Demux/1 -> Gain4/1, Mux3/2  "wx"
  Gain4/1 -> Mux2/3
  Mux1/1 -> Matrix Concatenate1/1
  Mux2/1 -> Matrix Concatenate1/2
  Gain5/1 -> Mux3/1
  Constant/1 -> Mux1/1
  Mux3/1 -> Matrix Concatenate1/3
  w(t)/1 -> Demux/1

== system uncontrolled_group24/Kinematics_DCM/Subsystem ==
  In1 : Inport
  Matrix Multiply : Product  Multiplication=Matrix(*)
  Matrix Multiply1 : Product  Multiplication=Matrix(*)
  Multiply : Gain  Gain=3/2
  Multiply1 : Gain  Gain=1/2
  Subtract : Sum  Inputs=+-
  Transpose : Math  Operator=transpose
  Out2 : Outport
  wires:
  Subtract/1 -> Out2/1
  Multiply1/1 -> Subtract/2
  Matrix Multiply1/1 -> Multiply1/1
  Multiply/1 -> Subtract/1
  Transpose/1 -> Matrix Multiply/2
  Matrix Multiply/1 -> Matrix Multiply1/1
  In1/1 -> Multiply/1, Transpose/1, Matrix Multiply1/2, Matrix Multiply/1  "A"

== system uncontrolled_group24/Sensors/Gyroscope ==
  note: w_BN_measured = G(w_B) A_eps w_BN + n + b
  w : Inport
  ARW : RandomNumber  Variance=(deg2rad(ARW)/sqrt(3600)/sqrt(1/GyroSampleRate))^2*[1;1;1]  SampleTime=1/GyroSampleRate
  Integrator : Integrator
  RRW : RandomNumber  Variance=(deg2rad(RRW)/3600/sqrt(1/GyroSampleRate))^2* [1;1;1]  SampleTime=1/GyroSampleRate
  Sum : Sum  Inputs=+++
  w_meas : Outport
  wires:
  RRW/1 -> Integrator/1  "b_dot"
  ARW/1 -> Sum/2  "n"
  Integrator/1 -> Sum/3  "b"
  Sum/1 -> w_meas/1
  w/1 -> Sum/1

== system uncontrolled_group24/Sensors/Magnetometer ==
  b_B : Inport
  Constant : Constant  Value=MMnoise
  MatrixMultiply : Product  Multiplication=Matrix(*)
  Subsystem : Subsystem
  Sum : Sum
  b_meas_B : Outport
  wires:
  Constant/1 -> Sum/2
  b_B/1 -> Sum/1  "b_B"
  Subsystem/1(A_epsMM) -> MatrixMultiply/1
  Sum/1 -> MatrixMultiply/2
  MatrixMultiply/1 -> b_meas_B/1

== system uncontrolled_group24/Sensors/Sun Sensor ==
  Sun_N : Inport
  Matrix Multiply1 : Product  Multiplication=Matrix(*)
  Subsystem : Subsystem
  Ssens_N : Outport
  wires:
  Sun_N/1 -> Matrix Multiply1/2
  Subsystem/1(A_eps) -> Matrix Multiply1/1  "A_eps"
  Matrix Multiply1/1 -> Ssens_N/1

== system uncontrolled_group24/errormeasure/IJK_error ==
  A_BN_estimated : Inport
  A_B_N_ea : Inport  Port=2
  I : Constant  Value=[1 0 0]'
  I_Error : Subsystem
  J : Constant  Value=[0 1 0]'
  J_Error : Subsystem
  K : Constant  Value=[0 0 1]'
  K_Error : Subsystem
  Degrees out : Outport
  Degrees out1 : Outport  Port=2
  Degrees out2 : Outport  Port=3
  wires:
  A_BN_estimated/1 -> K_Error/1(A_BN_estimated), I_Error/1(A_BN_estimated), J_Error/1(A_BN_estimated)
  A_B_N_ea/1 -> K_Error/3(A_B_N_ea), I_Error/3(A_B_N_ea), J_Error/3(A_B_N_ea)
  K/1 -> K_Error/2(K)
  J_Error/1(Degrees out) -> Degrees out1/1
  J/1 -> J_Error/2(J)
  I_Error/1(Degrees out) -> Degrees out/1
  K_Error/1(Degrees out) -> Degrees out2/1
  I/1 -> I_Error/2(I)

== system uncontrolled_group24/errormeasure/r_n_Error ==
  A_BN_estimated : Inport
  r_n : Inport  Port=2
  A_B_N_ea : Inport  Port=3
  Acos : Trigonometry  Operator=acos
  Dot Product : DotProduct  OutDataTypeStr=Inherit: Inherit via internal rule
  MatrixMultiply : Product  Multiplication=Matrix(*)
  MatrixMultiply1 : Product  Multiplication=Matrix(*)
  Normalize Vector : vrlib/Utilities/Normalize Vector  maxzero=0
  Normalize Vector1 : vrlib/Utilities/Normalize Vector  maxzero=0
  Radians to Degrees : simulink_extras/Transformations/Radians to Degrees
  Degrees out : Outport
  wires:
  MatrixMultiply1/1 -> Normalize Vector/1
  Dot Product/1 -> Acos/1
  r_n/1 -> MatrixMultiply1/2, MatrixMultiply/2
  Normalize Vector1/1 -> Dot Product/2
  Normalize Vector/1 -> Dot Product/1
  Acos/1 -> Radians to Degrees/1  "Theta_err"
  A_BN_estimated/1 -> MatrixMultiply1/1
  MatrixMultiply/1 -> Normalize Vector1/1
  A_B_N_ea/1 -> MatrixMultiply/1
  Radians to Degrees/1 -> Degrees out/1

== system uncontrolled_group24/Desturbances/External Torques/M_GG ==
  A_BL : Inport
  r : Inport  Port=2
  GG Torque1 : Subsystem
  "c1, c2, c3" : Subsystem
  M_GG1 : Outport
  wires:
  A_BL/1 -> "c1, c2, c3"/1(A_BL)
  "c1, c2, c3"/1(c1) -> GG Torque1/1(c1)
  "c1, c2, c3"/2(c2) -> GG Torque1/2(c2)
  "c1, c2, c3"/3(c3) -> GG Torque1/3(c3)
  r/1 -> GG Torque1/4(r)
  GG Torque1/1(M_GG) -> M_GG1/1

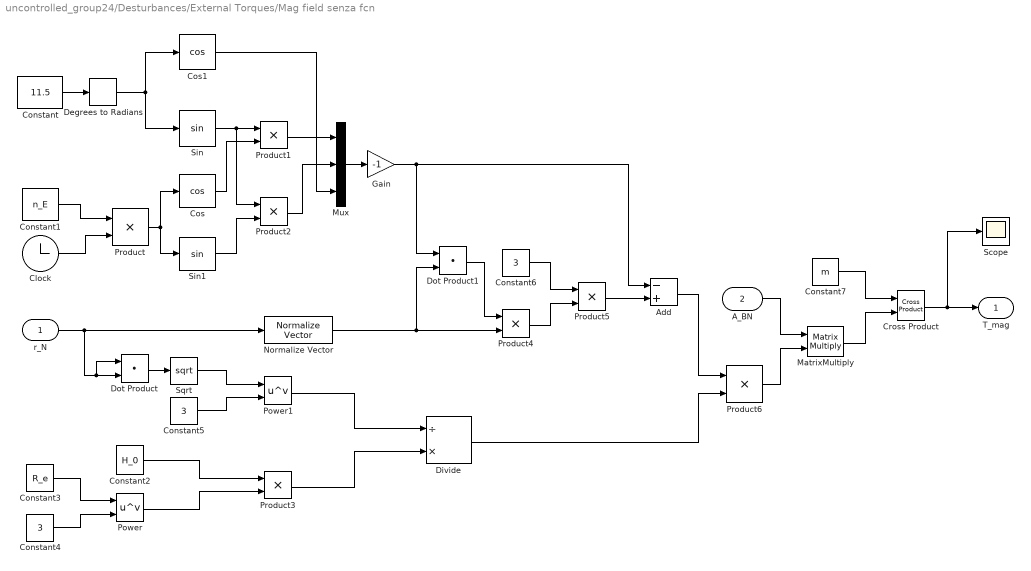
== system uncontrolled_group24/Desturbances/External Torques/Mag field senza fcn ==
  r_N : Inport
  A_BN : Inport  Port=2
  Add : Sum  Inputs=-+
  Clock : Clock
  Constant : Constant  Value=11.5
  Constant1 : Constant  Value=n_E
  Constant2 : Constant  Value=H_0
  Constant3 : Constant  Value=R_e
  Constant4 : Constant  Value=3
  Constant5 : Constant  Value=3
  Constant6 : Constant  Value=3
  Constant7 : Constant  Value=m
  Cos : Trigonometry  Operator=cos
  Cos1 : Trigonometry  Operator=cos
  Cross Product : vrlib/Utilities/Cross Product
  Degrees to Radians : simulink_extras/Transformations/Degrees to Radians
  Divide : Product  Inputs=/*
  Dot Product : DotProduct  OutDataTypeStr=Inherit: Inherit via internal rule
  Dot Product1 : DotProduct  OutDataTypeStr=Inherit: Inherit via internal rule
  Gain : Gain  Gain=-1
  MatrixMultiply : Product  Multiplication=Matrix(*)
  Mux : Mux  Inputs=3
  Normalize Vector : vrlib/Utilities/Normalize Vector  maxzero=0
  Power : Math  Operator=pow
  Power1 : Math  Operator=pow
  Product{,1..6} (7 alike) : Product
  Scope : Scope
  Sin : Trigonometry
  Sin1 : Trigonometry
  Sqrt : Sqrt
  T_mag : Outport
  wires:
  Constant/1 -> Degrees to Radians/1
  Constant1/1 -> Product/1
  Clock/1 -> Product/2
  Product/1 -> Sin1/1, Cos/1
  Sin/1 -> Product2/1, Product1/1
  Cos/1 -> Product1/2
  Sin1/1 -> Product2/2
  Product1/1 -> Mux/1
  Cos1/1 -> Mux/3
  Product2/1 -> Mux/2
  Constant4/1 -> Power/2
  Constant3/1 -> Power/1
  Constant5/1 -> Power1/2
  Constant2/1 -> Product3/1
  Power/1 -> Product3/2
  r_N/1 -> Dot Product/2, Dot Product/1, Normalize Vector/1
  Dot Product/1 -> Sqrt/1
  Sqrt/1 -> Power1/1
  Mux/1 -> Gain/1
  Normalize Vector/1 -> Product4/2, Dot Product1/2
  Dot Product1/1 -> Product4/1
  Constant6/1 -> Product5/1
  Product4/1 -> Product5/2
  Product6/1 -> MatrixMultiply/2
  A_BN/1 -> MatrixMultiply/1
  MatrixMultiply/1 -> Cross Product/2
  Constant7/1 -> Cross Product/1
  Cross Product/1 -> Scope/1, T_mag/1
  Product5/1 -> Add/2
  Power1/1 -> Divide/1
  Product3/1 -> Divide/2
  Add/1 -> Product6/1
  Divide/1 -> Product6/2
  Degrees to Radians/1 -> Cos1/1, Sin/1
  Gain/1 -> Dot Product1/1, Add/1

== system uncontrolled_group24/Desturbances/External Torques/Magnetic field ==
  r_L : Inport
  A_BN : Inport  Port=2
  Clock : Clock
  Constant : Constant  Value=m
  Constant1 : Constant  Value=R_e*1000
  Constant3 : Constant  Value=G
  Constant4 : Constant  Value=H
  Cross Product1 : matrix_library/Cross Product
  MATLAB Function : MATLAB Function  TreatAsAtomicUnit=on
  MatrixMultiply : Product  Multiplication=Matrix(*)
  Reshape1 : Reshape  OutputDimensionality=Column vector (2-D)
  M_MAG : Outport
  b_B : Outport  Port=2
  wires:
  Constant1/1 -> MATLAB Function/2(r)
  Clock/1 -> MATLAB Function/3(t)
  Constant3/1 -> MATLAB Function/4(G)
  MATLAB Function/1(b_N) -> Reshape1/1
  r_L/1 -> MATLAB Function/1(r_LVLH)
  Reshape1/1 -> MatrixMultiply/2
  Constant4/1 -> MATLAB Function/5(H)
  A_BN/1 -> MatrixMultiply/1
  Constant/1 -> Cross Product1/1
  MatrixMultiply/1 -> b_B/1, Cross Product1/2
  Cross Product1/1 -> M_MAG/1

== system uncontrolled_group24/Desturbances/External Torques/SRP con frecce ==
  r_s_B : Inport
  Normalize Vector : vrlib/Utilities/Normalize Vector  maxzero=0
  SRP : Subsystem
  Tsrp : Outport
  wires:
  r_s_B/1 -> Normalize Vector/1
  Normalize Vector/1 -> SRP/1(r_s_B)
  SRP/1(Tsrp) -> Tsrp/1
